simulink model "PID"  (R2023a)
settings: Solver=VariableStepAuto  StartTime=0.0  StopTime=1  RelTol=1e-3
undefined symbols (not defined in the file): kip, kpd, kpid
settings Model: Creator=manui  LastModifiedBy=manui

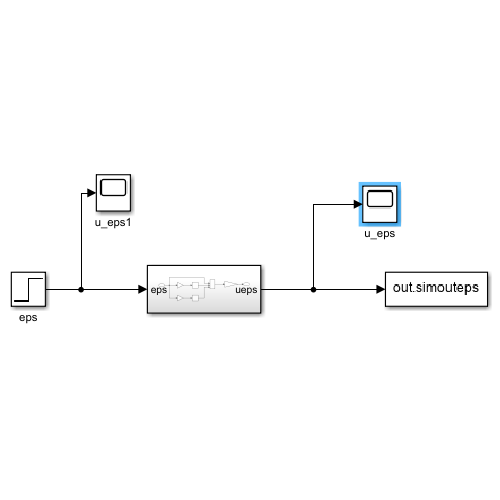
[thumbnail: Simulink's stored preview of the top-level diagram]
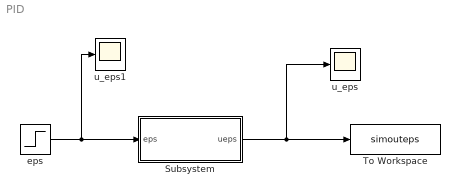
== system PID ==
  Subsystem : Subsystem
  To Workspace : ToWorkspace  VariableName=simouteps  SaveFormat=Timeseries  SampleTime=-1
  eps : Step  Time=0.1  SampleTime=0
  u_eps : Scope
  u_eps1 : Scope
  wires:
  eps/1 -> u_eps1/1, Subsystem/1(eps)
  Subsystem/1(ueps) -> u_eps/1, To Workspace/1

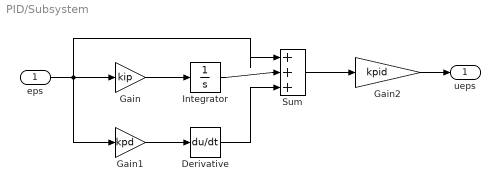
== system PID/Subsystem ==
  eps : Inport
  Derivative : Derivative
  Gain : Gain  Gain=kip
  Gain1 : Gain  Gain=kpd
  Gain2 : Gain  Gain=kpid
  Integrator : Integrator
  Sum : Sum  Inputs=|+++
  ueps : Outport
  wires:
  eps/1 -> Gain1/1, Sum/1, Gain/1
  Gain/1 -> Integrator/1
  Integrator/1 -> Sum/2
  Gain1/1 -> Derivative/1
  Derivative/1 -> Sum/3
  Sum/1 -> Gain2/1
  Gain2/1 -> ueps/1
